simulink model "Transitions7_2018a"  (R2018a)
settings: Solver=VariableStepAuto  StartTime=0.0  StopTime=0.1  RelTol=1e-3
settings Model: Creator=BEAR  LastModifiedBy=bzhan

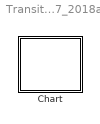
== system Transitions7_2018a ==
  Chart : Stateflow chart  TreatAsAtomicUnit=on

== stateflow chart Transitions7_2018a/Chart ==
  settings: updateMethod=DISCRETE  sampleTime=0.1
  state S
    en: f("enS")
    du: f("duS")
    S -> S [order 1] : {f("ca")}/{f("ta")}
  state T
    en: f("enT")
  (default) -> S : {x=1;}
  S -> T [order 1] : [x>0]
  data: s function_input; x local
  function f(s):
    | function f(s)
    |   fprintf(s+"\n");
